simulink model "Phase_voltages_per_switching_state_MPC_6Phase"  (R2022a)
settings: Solver=FixedStepDiscrete  StartTime=0.0  StopTime=10.0  RelTol=1e-3
values from neighbouring files (symbols this model uses):
  Rt = 1e-8    (= 1e-08)    [MPC_params.m]
  u_dc = 565    [MPC_params.m]
undefined symbols (not defined in the file or in its folder): f_c
libraries: simulink x2, hdlsllib x2
settings Model: DataTypeOverride=Off  Creator=Andre Merx  LastModifiedBy=Andre Merx
settings SolverCC: AlgebraicLoopSolver=TrustRegion
settings DataIOCC: LimitDataPoints=on  SaveOutput=off  SaveTime=off
settings OptimizationCC: BlockReduction=off  ConditionallyExecuteInputs=off  DefaultParameterBehavior=Inlined  LifeSpan=inf
settings DebuggingCC: AlgebraicLoopMsg=error  SingleTaskRateTransMsg=error  UnconnectedInputMsg=warning  UnconnectedOutputMsg=warning  UnconnectedLineMsg=warning  AllowSymbolicDim=off  StrictBusMsg=ErrorOnBusTreatedAsVector  SFUnexpectedBacktrackingDiag=warning  SFNoUnconditionalDefaultTransitionDiag=warning  SFExecutionAtInitializationDiag=none  SFMachineParentedDataDiag=warning  ArithmeticOperatorsInVariantConditions=warning
settings HardwareCC: ProdBitPerPointer=32  ProdBitPerSizeT=32  ProdBitPerPtrDiffT=32  ProdLargestAtomicFloat=None  ProdIntDivRoundTo=Undefined  ProdEndianess=Unspecified  ProdWordSize=32  ProdHWDeviceType=ASIC/FPGA->ASIC/FPGA  ProdEqTarget=off
settings SFSimCC: SimUseLocalCustomCode=off  CustomCodeUndefinedFunction=UseInterfaceOnly
settings RTWCC: RTWUseLocalCustomCode=off
settings CodeAppCC: StateflowObjectComments=on
settings GRTTargetCC: TargetLangStandard=C89/C90 (ANSI)
settings ConfigComp: CovScope=ReferencedModels  CovMetricSettings=dw  CovSaveCumulativeToWorkspaceVar=on  CovSaveSingleToWorkspaceVar=on  CovExternalEMLEnable=off  CovSFcnEnable=off

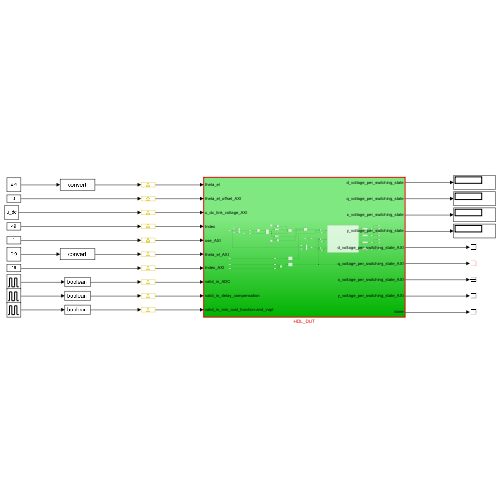
[thumbnail: Simulink's stored preview of the top-level diagram]
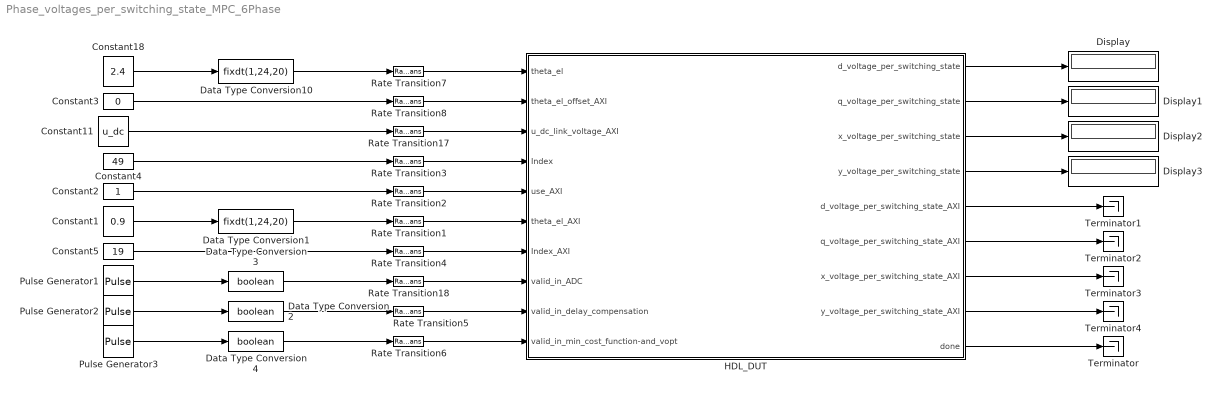
== system Phase_voltages_per_switching_state_MPC_6Phase ==
  Constant1 : Constant  Value=0.9
  Constant11 : Constant  Value=u_dc  OutDataTypeStr=single  SampleTime=-1
  Constant18 : Constant  Value=2.4
  Constant2 : Constant  OutDataTypeStr=boolean  SampleTime=-1
  Constant3 : Constant  Value=0  OutDataTypeStr=single  SampleTime=-1
  Constant4 : Constant  Value=49  OutDataTypeStr=int32  SampleTime=-1
  Constant5 : Constant  Value=19  OutDataTypeStr=int32  SampleTime=-1
  Data Type Conversion1 : DataTypeConversion  OutDataTypeStr=fixdt(1,24,20)  SaturateOnIntegerOverflow=off  RndMeth=Floor
  Data Type Conversion10 : DataTypeConversion  OutDataTypeStr=fixdt(1,24,20)  SaturateOnIntegerOverflow=off  RndMeth=Floor
  Data Type Conversion2 : DataTypeConversion  OutDataTypeStr=boolean  SaturateOnIntegerOverflow=off  RndMeth=Floor
  Data Type Conversion3 : DataTypeConversion  OutDataTypeStr=boolean  SaturateOnIntegerOverflow=off  RndMeth=Floor
  Data Type Conversion4 : DataTypeConversion  OutDataTypeStr=boolean  SaturateOnIntegerOverflow=off  RndMeth=Floor
  Display{,1..3} (4 alike) : Display
  HDL_DUT : Subsystem  TreatAsAtomicUnit=on
  Pulse Generator1 : DiscretePulseGenerator  PulseType=Time based  Period=1/f_c
  Pulse Generator2 : DiscretePulseGenerator  PulseType=Time based  Period=1/f_c
  Pulse Generator3 : DiscretePulseGenerator  PulseType=Time based  Period=1/f_c
  Rate Transition{1..8,17..18} (10 alike) : RateTransition  OutPortSampleTime=Rt
  Terminator{,1..4} (5 alike) : Terminator
  wires:
  Constant11/1 -> Rate Transition17/1
  Data Type Conversion10/1 -> Rate Transition7/1
  Rate Transition17/1 -> HDL_DUT/3(u_dc_link_voltage_AXI)
  Rate Transition7/1 -> HDL_DUT/1(theta_el)
  Constant3/1 -> Rate Transition8/1
  Constant18/1 -> Data Type Conversion10/1
  Rate Transition8/1 -> HDL_DUT/2(theta_el_offset_AXI)
  Pulse Generator1/1 -> Data Type Conversion3/1
  Data Type Conversion3/1 -> Rate Transition18/1
  Rate Transition18/1 -> HDL_DUT/8(valid_in_ADC)
  Data Type Conversion1/1 -> Rate Transition1/1
  Constant1/1 -> Data Type Conversion1/1
  Rate Transition1/1 -> HDL_DUT/6(theta_el_AXI)
  Constant2/1 -> Rate Transition2/1
  Rate Transition2/1 -> HDL_DUT/5(use_AXI)
  HDL_DUT/1(d_voltage_per_switching_state) -> Display/1
  HDL_DUT/2(q_voltage_per_switching_state) -> Display1/1
  HDL_DUT/3(x_voltage_per_switching_state) -> Display2/1
  HDL_DUT/4(y_voltage_per_switching_state) -> Display3/1
  Constant4/1 -> Rate Transition3/1
  Rate Transition3/1 -> HDL_DUT/4(Index)
  Constant5/1 -> Rate Transition4/1
  Rate Transition4/1 -> HDL_DUT/7(Index_AXI)
  HDL_DUT/5(d_voltage_per_switching_state_AXI) -> Terminator1/1
  HDL_DUT/6(q_voltage_per_switching_state_AXI) -> Terminator2/1
  HDL_DUT/7(x_voltage_per_switching_state_AXI) -> Terminator3/1
  HDL_DUT/8(y_voltage_per_switching_state_AXI) -> Terminator4/1
  Pulse Generator2/1 -> Data Type Conversion2/1
  Data Type Conversion2/1 -> Rate Transition5/1
  Rate Transition5/1 -> HDL_DUT/9(valid_in_delay_compensation)
  Pulse Generator3/1 -> Data Type Conversion4/1
  Data Type Conversion4/1 -> Rate Transition6/1
  Rate Transition6/1 -> HDL_DUT/10(valid_in_min_cost_function-and_vopt)
  HDL_DUT/9(done) -> Terminator/1

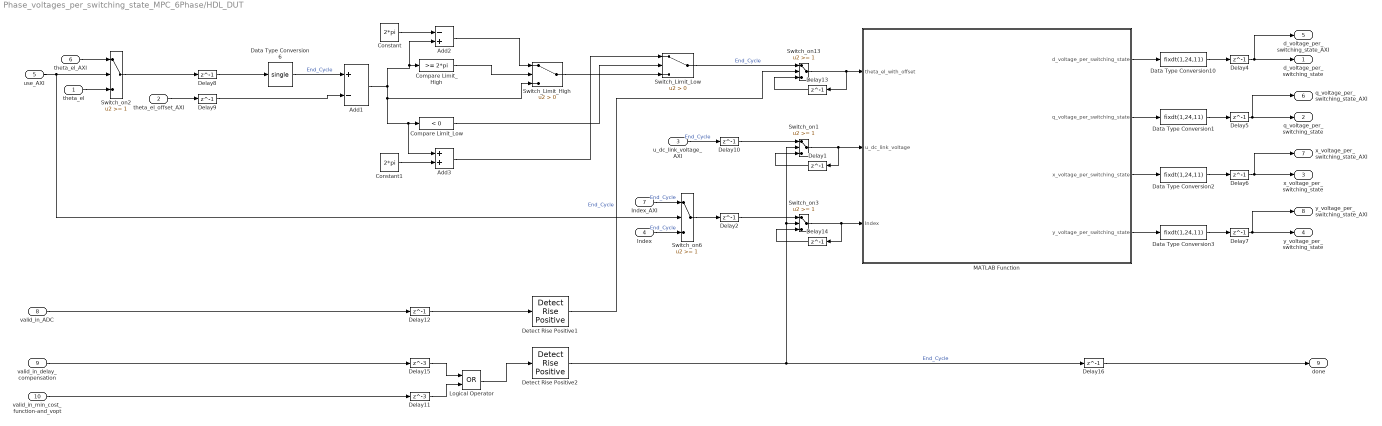
== system Phase_voltages_per_switching_state_MPC_6Phase/HDL_DUT ==
  theta_el : Inport
  theta_el_offset_AXI : Inport  Port=2
  u_dc_link_voltage_AXI : Inport  Port=3
  Index : Inport  Port=4
  use_AXI : Inport  Port=5
  theta_el_AXI : Inport  Port=6
  Index_AXI : Inport  Port=7
  valid_in_ADC : Inport  Port=8
  valid_in_delay_compensation : Inport  Port=9
  valid_in_min_cost_function-and_vopt : Inport  Port=10
  Add1 : Sum  Inputs=+-  OutDataTypeStr=Inherit: Same as accumulator
  Add2 : Sum  Inputs=-+  OutDataTypeStr=Inherit: Same as first input
  Add3 : Sum  OutDataTypeStr=Inherit: Same as first input
  Compare Limit_High : simulink/Logic and Bit Operations/Compare To Constant  relop=>=  const=2*pi  OutDataTypeStr=boolean
  Compare Limit_Low : simulink/Logic and Bit Operations/Compare To Constant  relop=<  const=0  OutDataTypeStr=boolean
  Constant : Constant  Value=2*pi  OutDataTypeStr=single  SampleTime=Rt
  Constant1 : Constant  Value=2*pi  OutDataTypeStr=single  SampleTime=Rt
  Data Type Conversion{1..3,10} (4 alike) : DataTypeConversion  OutDataTypeStr=fixdt(1,24,11)  SaturateOnIntegerOverflow=off  RndMeth=Floor
  Data Type Conversion6 : DataTypeConversion  OutDataTypeStr=single  RndMeth=Nearest  SaturateOnIntegerOverflow=off
  Delay{1..2,4..10,12..14,16} (13 alike) : Delay  DelayLength=1
  Delay11 : Delay  DelayLength=3
  Delay15 : Delay  DelayLength=3
  Detect Rise Positive1 : hdlsllib/Logic and Bit Operations/Detect Rise Positive  vinit=0  OutDataTypeStr=boolean
      settings: SourceProductBaseCode=SL
  Detect Rise Positive2 : hdlsllib/Logic and Bit Operations/Detect Rise Positive  vinit=0  OutDataTypeStr=boolean
      settings: SourceProductBaseCode=SL
  Logical Operator : Logic  Operator=OR  AllPortsSameDT=off  OutDataTypeStr=boolean
  MATLAB Function : MATLAB Function  TreatAsAtomicUnit=on
  Switch_Limit_High : Switch  Criteria=u2 > Threshold  OutDataTypeStr=single  SaturateOnIntegerOverflow=off  InputSameDT=off
  Switch_Limit_Low : Switch  Criteria=u2 > Threshold  OutDataTypeStr=single  SaturateOnIntegerOverflow=off  InputSameDT=off
  Switch_on1 : Switch  Threshold=1  OutDataTypeStr=single  RndMeth=Simplest  SaturateOnIntegerOverflow=off  InputSameDT=off
  Switch_on13 : Switch  Threshold=1  OutDataTypeStr=single  RndMeth=Simplest  SaturateOnIntegerOverflow=off  InputSameDT=off
  Switch_on2 : Switch  Threshold=1  OutDataTypeStr=Inherit: Inherit via back propagation  RndMeth=Simplest  SaturateOnIntegerOverflow=off  InputSameDT=off
  Switch_on3 : Switch  Threshold=1  OutDataTypeStr=Inherit: Inherit via back propagation  RndMeth=Simplest  SaturateOnIntegerOverflow=off  InputSameDT=off
  Switch_on6 : Switch  Threshold=1  OutDataTypeStr=Inherit: Inherit via back propagation  RndMeth=Simplest  SaturateOnIntegerOverflow=off  InputSameDT=off
  d_voltage_per_switching_state : Outport
  q_voltage_per_switching_state : Outport  Port=2
  x_voltage_per_switching_state : Outport  Port=3
  y_voltage_per_switching_state : Outport  Port=4
  d_voltage_per_switching_state_AXI : Outport  Port=5
  q_voltage_per_switching_state_AXI : Outport  Port=6
  x_voltage_per_switching_state_AXI : Outport  Port=7
  y_voltage_per_switching_state_AXI : Outport  Port=8
  done : Outport  Port=9
  wires:
  MATLAB Function/4(y_voltage_per_switching_state) -> Data Type Conversion3/1
  Delay8/1 -> Data Type Conversion6/1
  Compare Limit_High/1 -> Switch_Limit_High/2
  MATLAB Function/2(q_voltage_per_switching_state) -> Data Type Conversion1/1
  Delay14/1 -> Switch_on3/3
  Delay7/1 -> y_voltage_per_switching_state/1, y_voltage_per_switching_state_AXI/1
  Delay13/1 -> Switch_on13/3
  Switch_on13/1 -> Delay13/1, MATLAB Function/1(theta_el_with_offset)
  u_dc_link_voltage_AXI/1 -> Delay10/1  "End_Cycle"
  theta_el_offset_AXI/1 -> Delay9/1
  Delay6/1 -> x_voltage_per_switching_state_AXI/1, x_voltage_per_switching_state/1
  Switch_Limit_High/1 -> Switch_Limit_Low/3
  Constant/1 -> Add2/1
  MATLAB Function/3(x_voltage_per_switching_state) -> Data Type Conversion2/1
  Delay10/1 -> Switch_on1/1
  Delay12/1 -> Detect Rise Positive1/1
  Delay9/1 -> Add1/2
  Add3/1 -> Switch_Limit_Low/1
  Delay5/1 -> q_voltage_per_switching_state/1, q_voltage_per_switching_state_AXI/1
  MATLAB Function/1(d_voltage_per_switching_state) -> Data Type Conversion10/1
  Data Type Conversion6/1 -> Add1/1  "End_Cycle"
  Switch_Limit_Low/1 -> Switch_on13/1  "End_Cycle"
  Add1/1 -> Switch_Limit_High/3, Add3/1, Compare Limit_Low/1, Add2/2, Compare Limit_High/1
  valid_in_ADC/1 -> Delay12/1
  Switch_on1/1 -> Delay1/1, MATLAB Function/2(u_dc_link_voltage)
  Compare Limit_Low/1 -> Switch_Limit_Low/2
  Switch_on3/1 -> Delay14/1, MATLAB Function/3(Index)
  Delay1/1 -> Switch_on1/3
  Constant1/1 -> Add3/2
  Delay4/1 -> d_voltage_per_switching_state_AXI/1, d_voltage_per_switching_state/1
  Add2/1 -> Switch_Limit_High/1
  theta_el/1 -> Switch_on2/3
  Switch_on2/1 -> Delay8/1
  theta_el_AXI/1 -> Switch_on2/1
  use_AXI/1 -> Switch_on6/2, Switch_on2/2
  Data Type Conversion10/1 -> Delay4/1
  Data Type Conversion1/1 -> Delay5/1
  Data Type Conversion2/1 -> Delay6/1
  Data Type Conversion3/1 -> Delay7/1
  Delay2/1 -> Switch_on3/1
  Switch_on6/1 -> Delay2/1
  Index/1 -> Switch_on6/3  "End_Cycle"
  Index_AXI/1 -> Switch_on6/1  "End_Cycle"
  valid_in_min_cost_function-and_vopt/1 -> Delay11/1
  Delay11/1 -> Logical Operator/2
  Logical Operator/1 -> Detect Rise Positive2/1
  valid_in_delay_compensation/1 -> Delay15/1
  Delay15/1 -> Logical Operator/1
  Delay16/1 -> done/1
  Detect Rise Positive2/1 -> Switch_on3/2, Switch_on1/2, Delay16/1  "End_Cycle"
  Detect Rise Positive1/1 -> Switch_on13/2  "End_Cycle"

== matlab function Phase_voltages_per_switching_state_MPC_6Phase/HDL_DUT/MATLAB Function ==
  data: theta_el_with_offset input; d_voltage_per_switching_state output; u_dc_link_voltage input; Index input; q_voltage_per_switching_state output; x_voltage_per_switching_state output; y_voltage_per_switching_state output
function [d_voltage_per_switching_state, q_voltage_per_switching_state, x_voltage_per_switching_state, y_voltage_per_switching_state] = fcn(theta_el_with_offset, u_dc_link_voltage, Index)
      
        % Initial condition
        Index = Index+1;
    
        % Swichtingstates factors alpha beta x y
        Factors_alpha_beta_x_y = single([0	    0.333333333333333	-0.166666666666667	 0.166666666666667	-0.166666666666667	 0.166666666666667	-0.333333333333333	0	 0.288675134594813	0.622008467928146	 0.122008467928146  	0.455341801261480	 0.122008467928146	 0.455341801261480	-0.0446581987385205  0.288675134594813	-0.288675134594813	0.0446581987385205	-0.455341801261480	-0.122008467928146	-0.455341801261480	-0.122008467928146	-0.622008467928146	-0.288675134594813	0	                0.333333333333333	-0.166666666666667  	0.166666666666667	-0.166666666666667	 0.166666666666667	 -0.333333333333333	0	                 0	                 0.333333333333333	-0.166666666666667	  0.166666666666667	    -0.166666666666667	  0.166666666666667	    -0.333333333333333	 0	                 0.288675134594813	 0.622008467928146	 0.122008467928146	 0.455341801261480	 0.122008467928146	 0.455341801261480	-0.0446581987385205  0.288675134594813	-0.288675134594813	 0.0446581987385205  -0.455341801261480	  -0.122008467928146	-0.455341801261480	-0.122008467928146	-0.622008467928146	-0.288675134594813	0	0.333333333333333	-0.166666666666667	 0.166666666666667	-0.166666666666667	 0.166666666666667	-0.333333333333333	0;
                                         0	    0                    0.288675134594813	 0.288675134594813	-0.288675134594813	-0.288675134594813	 0	                0	 0.166666666666667	0.166666666666667	 0.455341801261480  	0.455341801261480	-0.122008467928146	-0.122008467928146	 0.166666666666667	 0.166666666666667	 0.166666666666667	0.166666666666667	 0.455341801261480   0.455341801261480	-0.122008467928146	-0.122008467928146	 0.166666666666667	 0.166666666666667	0.333333333333333	0.333333333333333	 0.622008467928146	    0.622008467928146	 0.0446581987385205	 0.0446581987385205	  0.333333333333333	0.333333333333333	-0.333333333333333	-0.333333333333333	-0.0446581987385205	 -0.0446581987385205	-0.622008467928146	 -0.622008467928146	    -0.333333333333333	-0.333333333333333	-0.166666666666667	-0.166666666666667	 0.122008467928146	 0.122008467928146	-0.455341801261480	-0.455341801261480	-0.166666666666667	-0.166666666666667	-0.166666666666667	-0.166666666666667	  0.122008467928146	   0.122008467928146	-0.455341801261480	-0.455341801261480	-0.166666666666667	-0.166666666666667	0	0	                 0.288675134594813	 0.288675134594813	-0.288675134594813	-0.288675134594813	 0	                0;
                                         0	    0.333333333333333	-0.166666666666667	 0.166666666666667	-0.166666666666667	 0.166666666666667	-0.333333333333333	0	-0.288675134594813	0.0446581987385205	-0.455341801261480	   -0.122008467928146	-0.455341801261480	-0.122008467928146	-0.622008467928146	-0.288675134594813	 0.288675134594813	0.622008467928146	 0.122008467928146	 0.455341801261480   0.122008467928146	 0.455341801261480	-0.0446581987385205	 0.288675134594813	0	                0.333333333333333	-0.166666666666667	    0.166666666666667	-0.166666666666667	 0.166666666666667	 -0.333333333333333	0	                 0	                 0.333333333333333	-0.166666666666667	  0.166666666666667	    -0.166666666666667	  0.166666666666667	    -0.333333333333333	 0	                -0.288675134594813	 0.0446581987385205	-0.455341801261480	-0.122008467928146	-0.455341801261480	-0.122008467928146	-0.622008467928146	-0.288675134594813	 0.288675134594813	 0.622008467928146	  0.122008467928146	   0.455341801261480	 0.122008467928146	 0.455341801261480	-0.0446581987385205  0.288675134594813	0	0.333333333333333	-0.166666666666667	 0.166666666666667	-0.166666666666667	 0.166666666666667	-0.333333333333333	0;
                                         0	    0	                -0.288675134594813	-0.288675134594813	 0.288675134594813	 0.288675134594813	 0              	0	 0.166666666666667	0.166666666666667	-0.122008467928146     -0.122008467928146	 0.455341801261480	 0.455341801261480	 0.166666666666667	 0.166666666666667	 0.166666666666667	0.166666666666667	-0.122008467928146	-0.122008467928146	 0.455341801261480	 0.455341801261480	 0.166666666666667	 0.166666666666667	0.333333333333333	0.333333333333333	 0.0446581987385205 	0.0446581987385205	 0.622008467928146	 0.622008467928146	  0.333333333333333	0.333333333333333	-0.333333333333333	-0.333333333333333	-0.622008467928146	 -0.622008467928146	    -0.0446581987385205	 -0.0446581987385205	-0.333333333333333	-0.333333333333333	-0.166666666666667	-0.166666666666667	-0.455341801261480	-0.455341801261480	 0.122008467928146	 0.122008467928146	-0.166666666666667	-0.166666666666667	-0.166666666666667	-0.166666666666667	 -0.455341801261480	  -0.455341801261480	 0.122008467928146	 0.122008467928146	-0.166666666666667	-0.166666666666667	0	0	                -0.288675134594813	-0.288675134594813	 0.288675134594813	 0.288675134594813	 0	                0]);
        
        % Park-Transformation of the switchingstates factors
        Factors_d_q_x_y =single(zeros(4,1));
    
        Factors_d_q_x_y(3,1) = Factors_alpha_beta_x_y(3,Index);
        Factors_d_q_x_y(4,1) = Factors_alpha_beta_x_y(4,Index);
    
        cos_theta_el = single(cos(theta_el_with_offset));
        sin_theta_el = single(sin(theta_el_with_offset));
       
        Factors_d_q_x_y(1,1) = cos_theta_el*Factors_alpha_beta_x_y(1,Index)+sin_theta_el*Factors_alpha_beta_x_y(2,Index);
        Factors_d_q_x_y(2,1) = -sin_theta_el*Factors_alpha_beta_x_y(1,Index)+cos_theta_el*Factors_alpha_beta_x_y(2,Index);
    
        %Calculation of the voltages per switching state in alpha beta coordinates
        d_q_x_y_voltages_per_switching_state = single(u_dc_link_voltage*Factors_d_q_x_y);
    
        d_voltage_per_switching_state = d_q_x_y_voltages_per_switching_state(1,1);
        q_voltage_per_switching_state = d_q_x_y_voltages_per_switching_state(2,1);
        x_voltage_per_switching_state = d_q_x_y_voltages_per_switching_state(3,1);
        y_voltage_per_switching_state = d_q_x_y_voltages_per_switching_state(4,1);
    

end
